simulink model "human_transpoter_systemModel_R2024a"  (R2024a)
settings: Solver=VariableStepAuto  StartTime=0.0  StopTime=10.0  RelTol=1e-3
values from neighbouring files (symbols this model uses):
  beta = 0.1    [Simulink_Task4_matlab.m]    (also in get_working_vals.m = -0.18; loop.m = 11; loop_test.m = 0.25; task_4.m = -0.18)
  C1 = M + Ig_w/R^2 + Mu    (= 102.24000248)    [Simulink_Task4_matlab.m]    (also in get_working_vals.m; loop.m; loop_test.m; task_4.m)
  C2 = 1/C2_    (= 0.0151515151515)    [Simulink_Task4_matlab.m]    (also in get_working_vals.m = 66; loop.m; loop_test.m; task_4.m = 66)
  C4 = Mu * Lg^2 + Ig_u    (= 86)    [Simulink_Task4_matlab.m]    (also in get_working_vals.m; loop.m; loop_test.m; task_4.m)
  C5 = C2    (= 0.0151515151515)    [Simulink_Task4_matlab.m]    (also in get_working_vals.m = 66; loop.m; loop_test.m; task_4.m = 66)
  Ft = 0    [Simulink_Task4_matlab.m]    (also in get_working_vals.m = 500; loop.m = 5; loop_test.m = 5; task_4.m = 1000)
  g = 9.81    [Simulink_Task4_matlab.m]    (also in get_working_vals.m; loop.m; loop_test.m; task_4.m)
  Lg = 1    [Simulink_Task4_matlab.m]    (also in get_working_vals.m; loop.m; loop_test.m; task_4.m)
  Mu = 66    [Simulink_Task4_matlab.m]    (also in get_working_vals.m; loop.m; loop_test.m; task_4.m)
settings Model: Creator=gabsk  LastModifiedBy=Arya Peer

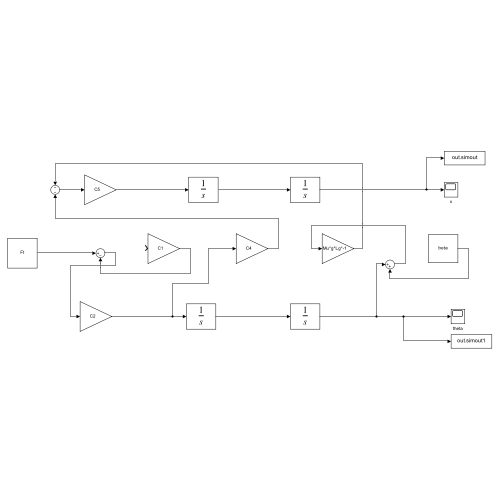
[thumbnail: Simulink's stored preview of the top-level diagram]
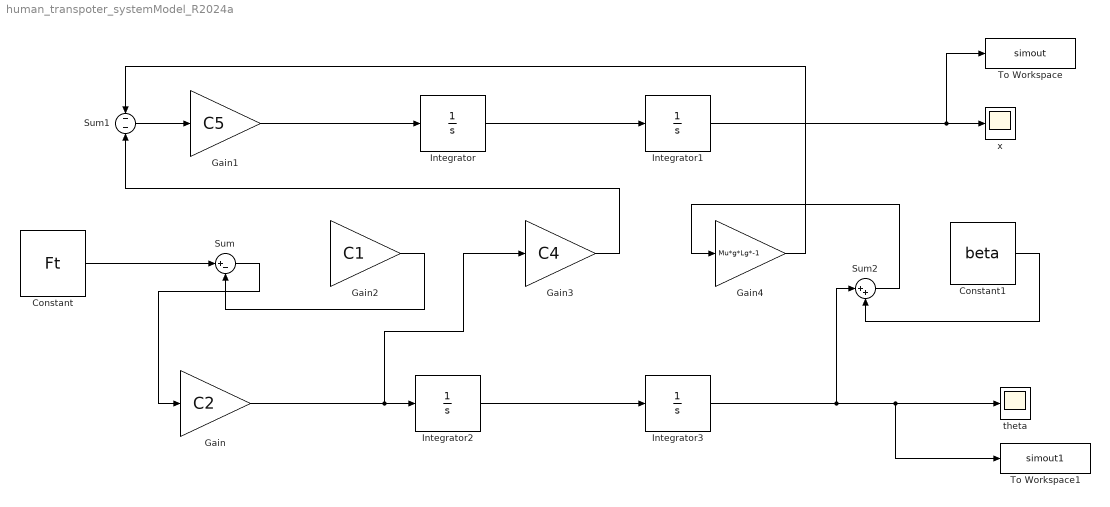
== system human_transpoter_systemModel_R2024a ==
  Constant : Constant  Value=Ft
  Constant1 : Constant  Value=beta
  Gain : Gain  Gain=C2
  Gain1 : Gain  Gain=C5
  Gain2 : Gain  Gain=C1
  Gain3 : Gain  Gain=C4
  Gain4 : Gain  Gain=Mu*g*Lg*-1
  Integrator{,1..3} (4 alike) : Integrator
  Sum : Sum  Inputs=|+-
  Sum1 : Sum  Inputs=--
  Sum2 : Sum  Inputs=|++
  To Workspace : ToWorkspace  VariableName=simout  SaveFormat=Structure With Time  SampleTime=-1
  To Workspace1 : ToWorkspace  VariableName=simout1  SaveFormat=Structure With Time  SampleTime=-1
  theta : Scope
  x : Scope
  wires:
  Integrator3/1 -> Sum2/1, To Workspace1/1, theta/1
  Integrator2/1 -> Integrator3/1
  Gain/1 -> Gain3/1, Integrator2/1
  Gain3/1 -> Sum1/2
  Gain2/1 -> Sum/2
  Constant/1 -> Sum/1
  Sum/1 -> Gain/1
  Sum1/1 -> Gain1/1
  Gain1/1 -> Integrator/1
  Integrator/1 -> Integrator1/1
  Integrator1/1 -> To Workspace/1, x/1
  Gain4/1 -> Sum1/1
  Constant1/1 -> Sum2/2
  Sum2/1 -> Gain4/1
